simulink model "Filtro_pasa_bajo_1er_orden"  (R2023b)
settings: Solver=VariableStepAuto  StartTime=0.0  StopTime=10.0  RelTol=1e-3
undefined symbols (not defined in the file): tau
settings Model: Creator=MSI  LastModifiedBy=MSI

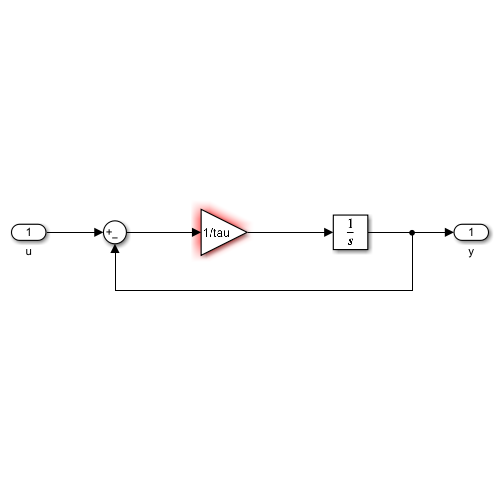
[thumbnail: Simulink's stored preview of the top-level diagram]
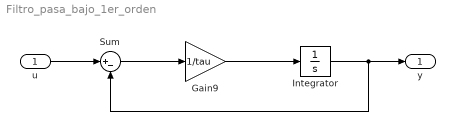
== system Filtro_pasa_bajo_1er_orden ==
  u : Inport
  Gain9 : Gain  Gain=1/tau
  Integrator : Integrator
  Sum : Sum  Inputs=|+-
  y : Outport
  wires:
  Sum/1 -> Gain9/1
  Gain9/1 -> Integrator/1
  u/1 -> Sum/1
  Integrator/1 -> Sum/2, y/1
